simulink model "hover"  (R2017a)
settings: Solver=VariableStepAuto  StartTime=0.0  StopTime=30  RelTol=1e-3
values from neighbouring files (symbols this model uses):
  J = 1    [setup_hover.m]
  K_LB = 1 * (0.95 + rand*0.1)    [setup_hover.m]
  K_LF = 1 * (0.95 + rand*0.1)    [setup_hover.m]
  K_RB = 1 * (0.95 + rand*0.1)    [setup_hover.m]
  K_RF = 1 * (0.95 + rand*0.1)    [setup_hover.m]
  m = 1    [setup_hover.m]
  T_LB = 1 * (0.95 + rand*0.1)    [setup_hover.m]
  T_LF = 1 * (0.95 + rand*0.1)    [setup_hover.m]
  T_RB = 1 * (0.95 + rand*0.1)    [setup_hover.m]
  T_RF = 1 * (0.95 + rand*0.1)    [setup_hover.m]
libraries: simulink x3
settings Model: Creator=cnjones  LastModifiedBy=cnjones

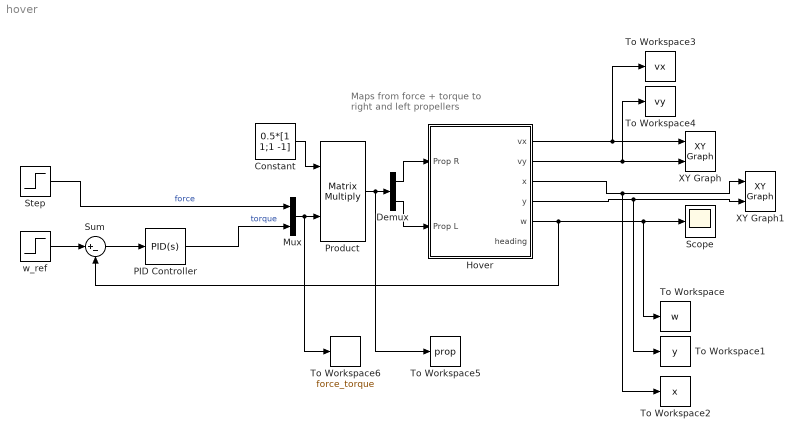
== system hover ==
  note: Maps from force + torque to
      | right and left propellers
  Constant : Constant  Value=0.5*[1 1;1 -1]
  Demux : Demux  Outputs=2
  Hover : Subsystem
  Mux : Mux  Inputs=2
  PID Controller : simulink/Continuous/PID Controller  Controller=PID  TimeDomain=Continuous-time  SampleTime=-1  IntegratorMethod=Forward Euler  FilterMethod=Forward Euler  Form=Ideal  UseFilter=on  ControllerParametersSource=internal  P=-1.30263726087134  I=1.05750099590497  D=0  N=100  InitialConditionSource=internal  InitialConditionForIntegrator=0  InitialConditionForFilter=0  ExternalReset=none  LimitOutput=off  UpperSaturationLimit=inf  LowerSaturationLimit=-inf  LinearizeAsGain=on  AntiWindupMode=none  Kb=1  TrackingMode=off  Kt=1  PParamMin=[]  PParamMax=[]  IParamMin=[]  IParamMax=[]  DParamMin=[]  DParamMax=[]  NParamMin=[]  NParamMax=[]  KbParamMin=[]  KbParamMax=[]  KtParamMin=[]  KtParamMax=[]  POutMin=[]  POutMax=[]  IOutMin=[]  IOutMax=[]  DOutMin=[]  DOutMax=[]  NOutMin=[]  NOutMax=[]  KbOutMin=[]  KbOutMax=[]  KtOutMin=[]  KtOutMax=[]  IntegratorOutMin=[]  IntegratorOutMax=[]  FilterOutMin=[]  FilterOutMax=[]  SumOutMin=[]  SumOutMax=[]  SumI1OutMin=[]  SumI1OutMax=[]  SumI2OutMin=[]  SumI2OutMax=[]  SumI3OutMin=[]  SumI3OutMax=[]  SumDOutMin=[]  SumDOutMax=[]  SaturationOutMin=[]  SaturationOutMax=[]  IntegratorContinuousStateAttributes=''  IntegratorStateMustResolveToSignalObject=off  IntegratorRTWStateStorageClass=Auto  FilterContinuousStateAttributes=''  FilterStateMustResolveToSignalObject=off  FilterRTWStateStorageClass=Auto  DifferentiatorICPrevScaledInput=0  DifferentiatorOutMin=[]  DifferentiatorOutMax=[]  InitialConditionSetting=State (most efficient)
  Product : Product  Multiplication=Matrix(*)
  Scope : Scope
  Step : Step  After=1.3  SampleTime=3
  Sum : Sum  Inputs=|+-
  To Workspace : ToWorkspace  VariableName=w  SaveFormat=Timeseries  SampleTime=-1
  To Workspace1 : ToWorkspace  VariableName=y  SaveFormat=Timeseries  SampleTime=-1
  To Workspace2 : ToWorkspace  VariableName=x  SaveFormat=Timeseries  SampleTime=-1
  To Workspace3 : ToWorkspace  VariableName=vx  SaveFormat=Timeseries  SampleTime=-1
  To Workspace4 : ToWorkspace  VariableName=vy  SaveFormat=Timeseries  SampleTime=-1
  To Workspace5 : ToWorkspace  VariableName=prop  SaveFormat=Timeseries  SampleTime=-1
  To Workspace6 : ToWorkspace  VariableName=force_torque  SaveFormat=Timeseries  SampleTime=-1
  XY Graph : simulink/Sinks/XY Graph  xmin=-2  xmax=2  ymin=-2  ymax=2  st=-1
  XY Graph1 : simulink/Sinks/XY Graph  xmin=-10  xmax=10  ymin=-10  ymax=10  st=-1
  w_ref : Step  After=-1  SampleTime=0
  wires:
  Hover/5(w) -> Sum/2, To Workspace/1, Scope/1
  Hover/1(vx) -> To Workspace3/1, XY Graph/1
  Hover/2(vy) -> To Workspace4/1, XY Graph/2
  Constant/1 -> Product/1
  Step/1 -> Mux/1  "force"
  Mux/1 -> To Workspace6/1, Product/2
  Product/1 -> To Workspace5/1, Demux/1
  Demux/1 -> Hover/1(Prop R)
  Demux/2 -> Hover/2(Prop L)
  w_ref/1 -> Sum/1
  Sum/1 -> PID Controller/1
  PID Controller/1 -> Mux/2  "torque"
  Hover/3(x) -> To Workspace2/1, XY Graph1/1
  Hover/4(y) -> To Workspace1/1, XY Graph1/2

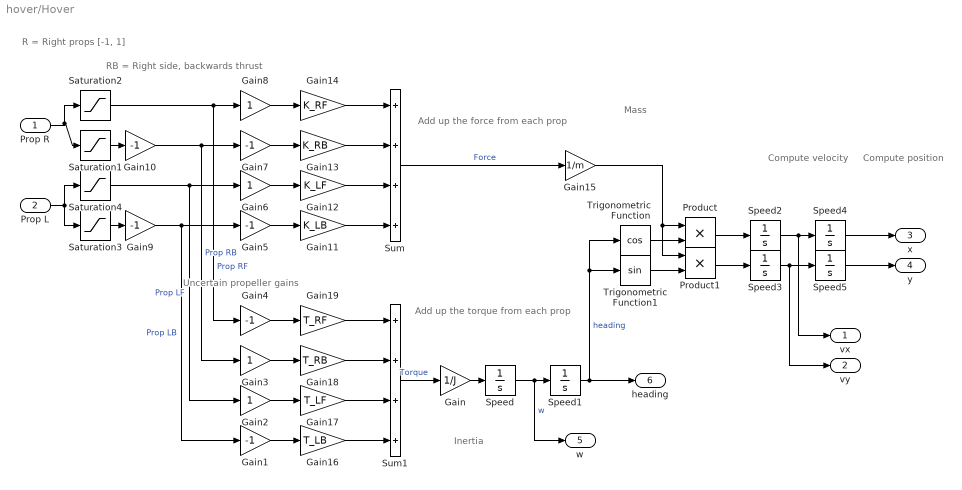
== system hover/Hover ==
  note: Mass
  note: Uncertain
      | propeller
      | gains
  note: Compute position
  note: Inertia
  note: R = Right props [-1, 1]
  note: RB = Right side, backwards thrust
  note: Compute velocity
  note: Add up the torque from each prop
  note: Add up the force from each prop
  Prop R : Inport
  Prop L : Inport  Port=2
  Gain : Gain  Gain=1/J
  Gain{1,4..5,7,9..10} (6 alike) : Gain  Gain=-1
  Gain11 : Gain  Gain=K_LB
  Gain12 : Gain  Gain=K_LF
  Gain13 : Gain  Gain=K_RB
  Gain14 : Gain  Gain=K_RF
  Gain15 : Gain  Gain=1/m
  Gain16 : Gain  Gain=T_LB
  Gain17 : Gain  Gain=T_LF
  Gain18 : Gain  Gain=T_RB
  Gain19 : Gain  Gain=T_RF
  Gain{2..3,6,8} (4 alike) : Gain
  Product : Product
  Product1 : Product
  Saturation1 : Saturate  UpperLimit=0  LowerLimit=-1
  Saturation2 : Saturate  UpperLimit=1  LowerLimit=0
  Saturation3 : Saturate  UpperLimit=0  LowerLimit=-1
  Saturation4 : Saturate  UpperLimit=1  LowerLimit=0
  Speed{,1..5} (6 alike) : Integrator
  Sum : Sum  Inputs=++++
  Sum1 : Sum  Inputs=++++
  Trigonometric Function : Trigonometry  Operator=cos
  Trigonometric Function1 : Trigonometry
  vx : Outport
  vy : Outport  Port=2
  x : Outport  Port=3
  y : Outport  Port=4
  w : Outport  Port=5
  heading : Outport  Port=6
  wires:
  Sum/1 -> Gain15/1  "Force"
  Gain/1 -> Speed/1
  Speed/1 -> w/1, Speed1/1  "w"
  Product1/1 -> Speed3/1
  Speed3/1 -> vy/1, Speed5/1
  Speed2/1 -> vx/1, Speed4/1
  Speed4/1 -> x/1
  Trigonometric Function1/1 -> Product1/2
  Trigonometric Function/1 -> Product/2
  Product/1 -> Speed2/1
  Saturation2/1 -> Gain4/1, Gain8/1  "Prop RF"
  Sum1/1 -> Gain/1  "Torque"
  Saturation4/1 -> Gain2/1, Gain6/1  "Prop LF"
  Speed1/1 -> heading/1, Trigonometric Function/1, Trigonometric Function1/1  "heading"
  Speed5/1 -> y/1
  Prop R/1 -> Saturation2/1, Saturation1/1
  Prop L/1 -> Saturation3/1, Saturation4/1
  Saturation3/1 -> Gain9/1
  Gain9/1 -> Gain1/1, Gain5/1  "Prop LB"
  Saturation1/1 -> Gain10/1
  Gain10/1 -> Gain3/1, Gain7/1  "Prop RB"
  Gain15/1 -> Product1/1, Product/1
  Gain14/1 -> Sum/1
  Gain8/1 -> Gain14/1
  Gain7/1 -> Gain13/1
  Gain6/1 -> Gain12/1
  Gain5/1 -> Gain11/1
  Gain13/1 -> Sum/2
  Gain12/1 -> Sum/3
  Gain11/1 -> Sum/4
  Gain4/1 -> Gain19/1
  Gain19/1 -> Sum1/1
  Gain3/1 -> Gain18/1
  Gain2/1 -> Gain17/1
  Gain1/1 -> Gain16/1
  Gain18/1 -> Sum1/2
  Gain17/1 -> Sum1/3
  Gain16/1 -> Sum1/4
